simulink model "fifth"  (R2020a)
settings: Solver=VariableStepAuto  StartTime=0.0  StopTime=10.0  RelTol=1e-3
model workspace (MAT data in the model file):
  C = Simulink.Parameter
  C.Value = 10
  C.DataType = 'auto'
  C.Dimensions = [1 1]
  R = Simulink.Parameter
  R.Value = 10
  R.DataType = 'auto'
  R.Dimensions = [1 1]
settings Model: Creator=Admin  LastModifiedBy=Admin

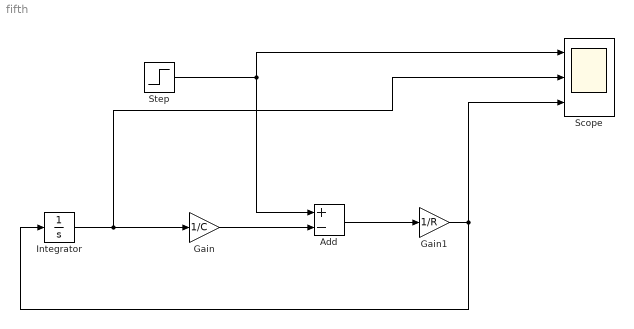
== system fifth ==
  Add : Sum  Inputs=+-
  Gain : Gain  Gain=1/C
  Gain1 : Gain  Gain=1/R
  Integrator : Integrator
  Scope : Scope  NumInputPorts=3
  Step : Step  SampleTime=0
  wires:
  Integrator/1 -> Scope/2, Gain/1
  Add/1 -> Gain1/1
  Gain1/1 -> Integrator/1, Scope/3
  Step/1 -> Scope/1, Add/1
  Gain/1 -> Add/2
